simulink model "uav_simulation_tarot"  (R2020a)
settings: Solver=VariableStepAuto  StartTime=0.0  StopTime=sim_params.max_sim_time  FixedStep=uav.dynamics_srate  MaxStep=uav.dynamics_srate  MinStep=.01  RelTol=1e-3
undefined symbols (not defined in the file): deg, DiscIntNeverNeededParam, processes, rad, s, sim_params, trajectory, uav
libraries: aerolibconvert2 x2, shared6dof x1
(part 1 of 2)
settings Model: Creator=Researcher  LastModifiedBy=darrahts
settings DataIOCC: ReturnWorkspaceOutputs=off
settings DebuggingCC: ArithmeticOperatorsInVariantConditions=warning
settings SFSimCC: SimUseLocalCustomCode=off  CustomCodeUndefinedFunction=UseInterfaceOnly
settings RTWCC: RTWUseLocalCustomCode=off

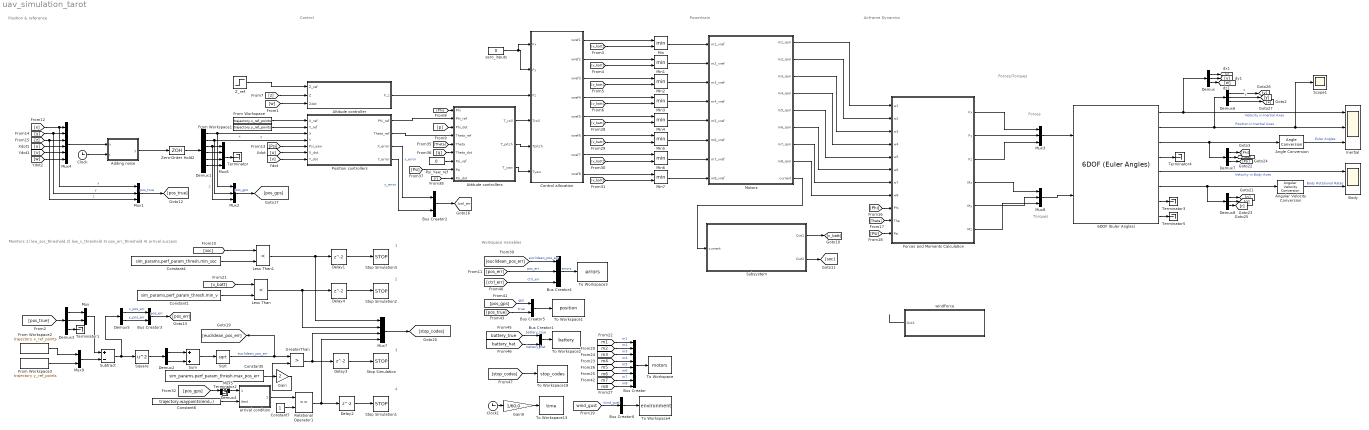
== system uav_simulation_tarot ==
  note: Airframe Dynamics
  note: 1
  note: Monitors
      | 	1) low_soc_threshold
      | 	2) low_v_threshold
      | 	3) pos_err_threshold
      | 	4) arrival success
  note: Powertrain
  note: Control
  note: 2
  note: 3
  note: 4
  note: Position & reference
  note: Workspace Variables
  note: Forces/Torques
  note: Torques
  note: Forces
  6DOF (Euler Angles) : shared6dof/6DOF (Euler Angles)  units=Metric (MKS)  mtype=Fixed  rep=Quaternion  xme_0=[sim_params.initial_conditions.X, sim_params.initial_conditions.Y, sim_params.initial_conditions.Z]  Vm_0=[0 0 0]  eul_0=[0 0 0]  pm_0=[0 0 0]  mass_0=uav.mass  mass_e=0.5  mass_f=2.0  inertia=uav.airframe.Jb  inertia_e=eye(3)  inertia_f=2*eye(3)  k_quat=1.0  vre_flag=on  abi_flag=off  aMode=0  xme_statename=''  Vm_statename=''  eul_statename=''  quat_statename=''  pm_statename=''  mass_statename=''
      settings: SourceProductBaseCode=AE,PW,MT,VE,VP
  Adding noise : MATLAB Function  TreatAsAtomicUnit=on  SystemSampleTime=uav.dynamics_srate
  Altitude controller : Subsystem
  Angle Conversion : aerolibconvert2/Angle Conversion  IU=rad  OU=deg
  Angular Velocity Conversion : aerolibconvert2/Angular Velocity Conversion  IU=rad/s  OU=deg/s
  Attitude controllers : Subsystem
  Body : Scope  NumInputPorts=2
  Bus Creator : BusCreator  Inputs=8
  Bus Creator{1..3,5} (4 alike) : BusCreator  Inputs=2
  Bus Creator4 : BusCreator  Inputs=3
  Bus Creator6 : BusCreator  Inputs=1
  Clock : Clock
  Clock1 : Clock
  Constant1 : Constant  Value=sim_params.perf_param_thresh.min_v
  Constant4 : Constant  Value=sim_params.perf_param_thresh.min_soc
  Constant5 : Constant  Value=sim_params.perf_param_thresh.max_pos_err
  Constant6 : Constant  Value=trajectory.waypoints(end,:)
  Constant7 : Constant
  Control allocation : MATLAB Function  TreatAsAtomicUnit=on
  Delay{1..4} (4 alike) : Delay
  Demux{,3..4,6..8} (6 alike) : Demux  Outputs=3
  Demux1 : Demux  Outputs=6
  Demux2 : Demux  Outputs=2
  Demux5 : Demux  Outputs=2
  Forces and Moments Calculation : MATLAB Function  TreatAsAtomicUnit=on
  From Workspace : FromWorkspace  VariableName=trajectory.x_ref_points  SampleTime=trajectory.sample_time
  From Workspace1 : FromWorkspace  VariableName=trajectory.y_ref_points  SampleTime=trajectory.sample_time
  From Workspace2 : FromWorkspace  VariableName=trajectory.x_ref_points  SampleTime=trajectory.sample_time
  From Workspace3 : FromWorkspace  VariableName=trajectory.y_ref_points  SampleTime=trajectory.sample_time
  Gain : Gain  Gain=2
  Gain9 : Gain  Gain=1/60.0
  GreaterThan : RelationalOperator  Operator=>  OutDataTypeStr=boolean  RndMeth=Simplest
  Inertial : Scope  NumInputPorts=3
  Less Than : RelationalOperator  Operator=<  OutDataTypeStr=boolean  RndMeth=Simplest
  Less Than1 : RelationalOperator  Operator=<  OutDataTypeStr=boolean  RndMeth=Simplest
  Min{,1..7} (8 alike) : MinMax  Inputs=2
  Motors : Subsystem
  Mux : Mux  Inputs=2
  Mux{1..3,8} (4 alike) : Mux  Inputs=3
  Mux4 : Mux  Inputs=6
  Mux5 : Mux  Inputs=2
  Mux6 : Mux
  Mux7 : Mux
  Mux9 : Mux  Inputs=2
  Position controllers : Subsystem
  Psi_Yaw_ref : Constant  Value=0
  Relational Operator1 : RelationalOperator  Operator===  OutDataTypeStr=boolean  RndMeth=Simplest
  Scope1 : Scope
  Sqrt : Sqrt  SaturateOnIntegerOverflow=on
  Square : Math  Operator=square  SaturateOnIntegerOverflow=on
  Stop Simulation{,1..3} (4 alike) : Stop
  Subsystem : Subsystem
  Subtract : Sum  Inputs=+-
  Sum : Sum
  Terminator{,1..5} (6 alike) : Terminator
  To Workspace : ToWorkspace  VariableName=motors  SaveFormat=Timeseries  SampleTime=-1
  To Workspace1 : ToWorkspace  VariableName=position  SaveFormat=Timeseries  SampleTime=-1
  To Workspace13 : ToWorkspace  VariableName=time  SaveFormat=Timeseries  SampleTime=-1
  To Workspace18 : ToWorkspace  VariableName=stop_codes  SaveFormat=Timeseries  SampleTime=-1
  To Workspace2 : ToWorkspace  VariableName=battery  SaveFormat=Timeseries  SampleTime=-1
  To Workspace3 : ToWorkspace  VariableName=errors  SaveFormat=Timeseries  SampleTime=-1
  To Workspace4 : ToWorkspace  VariableName=environment  SaveFormat=Timeseries  SampleTime=-1
  Z_ref : Step  Before=3  After=3  SampleTime=0
  Zero-Order Hold2 : ZeroOrderHold  SampleTime=uav.dynamics_srate
  arrival condition : MATLAB Function  TreatAsAtomicUnit=on
  windForce : Subsystem
  zero_inputs : Constant  Value=0
  wires:
  Clock/1 -> Adding noise/2(t)
  [y] -> Mux1/2, Mux4/2  "y"
  Zero-Order Hold2/1 -> Demux1/1
  [x] -> Mux1/1, Mux4/1  "x"
  [w] -> Mux4/6
  [z] -> Mux1/3, Mux4/3  "z"
  [v] -> Mux4/5
  [u] -> Mux4/4
  Mux4/1 -> Adding noise/1(u)
  Demux1/3 -> Mux2/3, Mux6/1  "z"
  Demux1/5 -> Mux6/3
  Demux1/4 -> Mux6/2
  Demux1/6 -> Mux6/4
  Demux1/2 -> Position controllers/4(Y), Mux2/2  "y"
  Demux1/1 -> Position controllers/3(X), Mux2/1  "x"
  Control allocation/6(wref6) -> Min5/1
  [v_batt] -> Min4/2
  Attitude controllers/1(T_roll) -> Control allocation/4(Troll)
  Min3/1 -> Motors/4(m4_vref)
  Position controllers/1(Phi_ref) -> Attitude controllers/2(Phi_ref)
  [r] -> Attitude controllers/9(Psi_dot)
  Z_ref/1 -> Altitude controller/1(Z_ref)
  [v_batt] -> Min3/2
  [v_batt] -> Min7/2
  Attitude controllers/3(T_yaw) -> Control allocation/6(Tyaw)
  Control allocation/8(wref8) -> Min7/1
  Bus Creator2/1 -> [ctrl_err]
  Min7/1 -> Motors/8(m8_vref)
  [Psi] -> Position controllers/5(Psi_yaw)
  [w] -> Altitude controller/3(Zdot)
  [u] -> Position controllers/6(X_dot)
  From Workspace/1 -> Position controllers/1(X_ref)
  Control allocation/7(wref7) -> Min6/1
  Position controllers/3(X_error) -> Bus Creator2/1  "x_error"
  Min2/1 -> Motors/3(m3_vref)
  Control allocation/3(wref3) -> Min2/1
  Min4/1 -> Motors/5(m5_vref)
  Attitude controllers/2(T_pitch) -> Control allocation/5(Tpitch)
  [Theta] -> Attitude controllers/5(Theta)
  Position controllers/2(Theta_ref) -> Attitude controllers/4(Theta_ref)
  Control allocation/1(wref1) -> Min/1
  Altitude controller/1(F_z) -> Control allocation/3(Fz)
  [Phi] -> Attitude controllers/1(Phi)
  [z] -> Altitude controller/2(Z)
  Position controllers/4(Y_error) -> Bus Creator2/2  "y_error"
  [v_batt] -> Min6/2
  Min5/1 -> Motors/6(m6_vref)
  Control allocation/4(wref4) -> Min3/1
  Min1/1 -> Motors/2(m2_vref)
  Control allocation/5(wref5) -> Min4/1
  Control allocation/2(wref2) -> Min1/1
  From Workspace1/1 -> Position controllers/2(Y_ref)
  [v] -> Position controllers/7(Y_dot)
  [Psi] -> Attitude controllers/8(Psi)
  Min6/1 -> Motors/7(m7_vref)
  zero_inputs/1 -> Control allocation/2(Fy), Control allocation/1(Fx)
  Min/1 -> Motors/1(m1_vref)
  [v_batt] -> Min/2
  [q] -> Attitude controllers/6(Theta_dot)
  Psi_Yaw_ref/1 -> Attitude controllers/7(Psi_ref)
  [p] -> Attitude controllers/3(Phi_dot)
  [v_batt] -> Min5/2
  [v_batt] -> Min1/2
  [v_batt] -> Min2/2
  Constant7/1 -> Relational Operator1/2
  Mux7/1 -> [stop_codes]
  Constant6/1 -> arrival condition/2(dest)
  Demux2/2 -> Sum/2
  Delay2/1 -> Stop Simulation1/1
  Constant5/1 -> Gain/1
  Gain9/1 -> To Workspace13/1
  arrival condition/1(arrived) -> Relational Operator1/1
  Demux2/1 -> Sum/1
  [pos_true] -> Demux3/1
  Mux9/1 -> Subtract/2
  Delay1/1 -> Stop Simulation3/1
  From Workspace3/1 -> Mux9/2
  Constant4/1 -> Less Than1/2
  Clock1/1 -> Gain9/1
  Sum/1 -> Sqrt/1
  [soc] -> Less Than1/1
  GreaterThan/1 -> Mux7/3, Delay3/1
  Sqrt/1 -> [euclidean_pos_err], GreaterThan/1  "euclidean_pos_err"
  Square/1 -> Demux2/1
  Subtract/1 -> Demux5/1, Square/1
  From Workspace2/1 -> Mux9/1
  [pos_gps] -> Demux4/1
  Relational Operator1/1 -> Mux7/4, Delay2/1
  Delay3/1 -> Stop Simulation/1
  Less Than1/1 -> Delay1/1, Mux7/1
  [stop_codes] -> To Workspace18/1
  [pos_gps] -> Bus Creator5/1  "gps"
  [battery_true] -> Bus Creator1/1  "battery_true"
  [battery_hat] -> Bus Creator1/2  "battery_hat"
  Motors/9(current) -> Subsystem/1(current)
  Subsystem/1(Out1) -> [v_batt]
  Subsystem/2(Out2) -> [soc]
  windForce/1(Out1) -> ?
  [m2] -> Bus Creator/2  "m2"
  Adding noise/1(y) -> Zero-Order Hold2/1
  Mux1/1 -> [pos_true]  "pos_true"
  Constant1/1 -> Less Than/2
  [v_batt] -> Less Than/1
  Delay4/1 -> Stop Simulation2/1
  Less Than/1 -> Mux7/2, Delay4/1
  [m1] -> Bus Creator/1  "m1"
  Bus Creator/1 -> To Workspace/1
  [m3] -> Bus Creator/3  "m3"
  [m4] -> Bus Creator/4  "m4"
  [m5] -> Bus Creator/5  "m5"
  [m6] -> Bus Creator/6  "m6"
  [m7] -> Bus Creator/7  "m7"
  [m8] -> Bus Creator/8  "m8"
  [pos_true] -> Bus Creator5/2  "true"
  Demux3/1 -> Mux/1
  Demux3/2 -> Mux/2
  Mux/1 -> Subtract/1
  Mux6/1 -> Terminator/1
  Mux2/1 -> [pos_gps]  "pos_gps"
  Demux3/3 -> Terminator1/1
  Demux4/1 -> Mux5/1
  Demux4/2 -> Mux5/2
  Mux5/1 -> arrival condition/1(currentpos)
  Demux4/3 -> Terminator2/1
  Bus Creator1/1 -> To Workspace2/1
  Demux5/1 -> Bus Creator3/1  "x_pos_err"
  Demux5/2 -> Bus Creator3/2  "y_pos_err"
  Bus Creator3/1 -> [pos_err]  "pos_err"
  [euclidean_pos_err] -> Bus Creator4/1  "euclidean_pos_err"
  [ctrl_err] -> Bus Creator4/3  "ctrl_err"
  [pos_err] -> Bus Creator4/2  "pos_err"
  Bus Creator4/1 -> To Workspace3/1  "errors"
  Bus Creator5/1 -> To Workspace1/1
  [wind_gust] -> Bus Creator6/1  "wind_gust"
  Bus Creator6/1 -> To Workspace4/1
  Gain/1 -> GreaterThan/2
  Forces and Moments Calculation/3(Fz) -> Mux3/3
  Forces and Moments Calculation/6(Mz) -> Mux8/3
  Angle Conversion/1 -> Inertial/3  "Euler Angles"
  Mux3/1 -> 6DOF (Euler Angles)/1
  Forces and Moments Calculation/5(My) -> Mux8/2
  Angular Velocity Conversion/1 -> Body/2  "Body Rotational Rates"
  Forces and Moments Calculation/2(Fy) -> Mux3/2
  Demux6/2 -> [y]  "y"
  Mux8/1 -> 6DOF (Euler Angles)/2
  6DOF (Euler Angles)/2 -> Demux6/1, Scope1/1, Inertial/2  "Position in Inertial Axes"
  Demux8/1 -> [p]
  Demux/3 -> [w]
  6DOF (Euler Angles)/8 -> Terminator5/1
  Demux6/1 -> [x]  "x"
  Demux7/2 -> [Theta]
  Forces and Moments Calculation/4(Mx) -> Mux8/1
  6DOF (Euler Angles)/7 -> Terminator3/1
  6DOF (Euler Angles)/6 -> Demux8/1, Angular Velocity Conversion/1
  Demux8/3 -> [r]
  Demux7/1 -> [Phi]
  Demux8/2 -> [q]
  6DOF (Euler Angles)/3 -> Demux7/1, Angle Conversion/1
  6DOF (Euler Angles)/4 -> Terminator4/1
  6DOF (Euler Angles)/1 -> Demux/1, Inertial/1  "Velocity in Inertial Axes"
  Demux6/3 -> [z]
  Forces and Moments Calculation/1(Fx) -> Mux3/1
  6DOF (Euler Angles)/5 -> Body/1  "Velocity in Body Axes"
  Demux7/3 -> [Psi]
  Demux/2 -> [v]
  Demux/1 -> [u]
  Motors/1(m1_rpm) -> Forces and Moments Calculation/1(w1)
  Motors/2(m2_rpm) -> Forces and Moments Calculation/2(w2)
  Motors/3(m3_rpm) -> Forces and Moments Calculation/3(w3)
  Motors/4(m4_rpm) -> Forces and Moments Calculation/4(w4)
  Motors/5(m5_rpm) -> Forces and Moments Calculation/5(w5)
  Motors/6(m6_rpm) -> Forces and Moments Calculation/6(w6)
  Motors/7(m7_rpm) -> Forces and Moments Calculation/7(w7)
  Motors/8(m8_rpm) -> Forces and Moments Calculation/8(w8)
  [Psi] -> Forces and Moments Calculation/11(Psi)
  [Theta] -> Forces and Moments Calculation/10(The)
  [Phi] -> Forces and Moments Calculation/9(Phi)

== system uav_simulation_tarot/Altitude controller ==
  Z_ref : Inport
  Z : Inport  Port=2
  Zdot : Inport  Port=3
  Add : Sum  Inputs=+++
  Add2 : Sum  Inputs=+-
  Constant2 : Constant  Value=9.8*uav.mass
  Kdz : Gain  Gain=-1
  Kpz : Gain  Gain=-0.5
  mass : Gain  Gain=uav.mass
  mass1 : Gain  Gain=uav.mass
  F_z : Outport  VectorParamsAs1DForOutWhenUnconnected=off
  wires:
  Add2/1 -> Kpz/1
  Constant2/1 -> Add/1
  Z/1 -> Add2/1
  Add/1 -> F_z/1
  Z_ref/1 -> Add2/2
  Zdot/1 -> Kdz/1
  Kpz/1 -> mass/1
  Kdz/1 -> mass1/1
  mass1/1 -> Add/3
  mass/1 -> Add/2

== system uav_simulation_tarot/Attitude controllers ==
  Phi : Inport
  Phi_ref : Inport  Port=2
  Phi_dot : Inport  Port=3
  Theta_ref : Inport  Port=4
  Theta : Inport  Port=5
  Theta_dot : Inport  Port=6
  Psi_ref : Inport  Port=7
  Psi : Inport  Port=8
  Psi_dot : Inport  Port=9
  PD_pitch : Subsystem
  PD_roll : Subsystem
  PD_yaw : Subsystem
  T_roll : Outport  VectorParamsAs1DForOutWhenUnconnected=off
  T_pitch : Outport  Port=2  VectorParamsAs1DForOutWhenUnconnected=off
  T_yaw : Outport  Port=3  VectorParamsAs1DForOutWhenUnconnected=off
  wires:
  PD_yaw/1(Tyaw) -> T_yaw/1
  PD_roll/1(Troll) -> T_roll/1
  Theta_ref/1 -> PD_pitch/1(Theta_ref)
  Theta_dot/1 -> PD_pitch/3(Theta_dot)
  PD_pitch/1(Tpitch) -> T_pitch/1
  Phi/1 -> PD_roll/2(Phi)
  Psi_dot/1 -> PD_yaw/3(Psi_dot)
  Psi_ref/1 -> PD_yaw/1(Psi_ref)
  Theta/1 -> PD_pitch/2(Theta)
  Phi_dot/1 -> PD_roll/3(Phi_dot)
  Psi/1 -> PD_yaw/2(Psi)
  Phi_ref/1 -> PD_roll/1(Phi_ref)

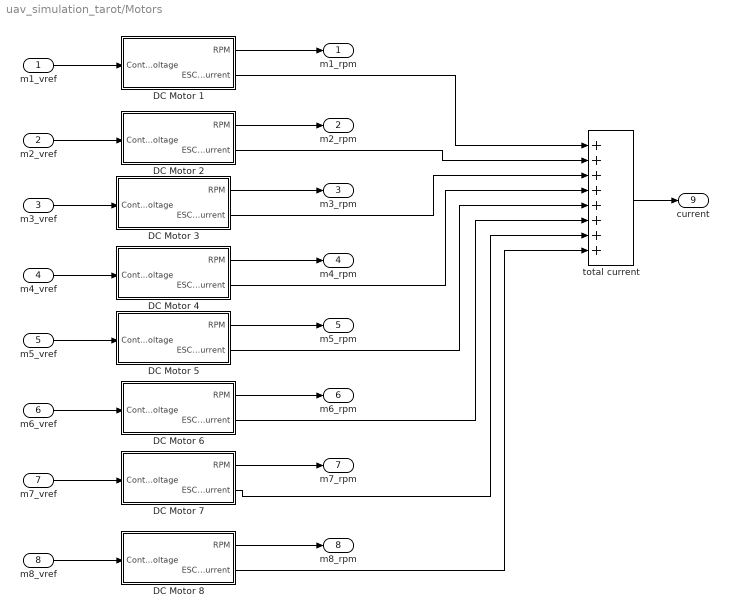
== system uav_simulation_tarot/Motors ==
  m1_vref : Inport
  m2_vref : Inport  Port=2
  m3_vref : Inport  Port=3
  m4_vref : Inport  Port=4
  m5_vref : Inport  Port=5
  m6_vref : Inport  Port=6
  m7_vref : Inport  Port=7
  m8_vref : Inport  Port=8
  DC Motor 1 : Subsystem
  DC Motor 2 : Subsystem
  DC Motor 3 : Subsystem
  DC Motor 4 : Subsystem
  DC Motor 5 : Subsystem
  DC Motor 6 : Subsystem
  DC Motor 7 : Subsystem
  DC Motor 8 : Subsystem
  total current : Sum  Inputs=++++++++
  m1_rpm : Outport  VectorParamsAs1DForOutWhenUnconnected=off
  m2_rpm : Outport  Port=2  VectorParamsAs1DForOutWhenUnconnected=off
  m3_rpm : Outport  Port=3  VectorParamsAs1DForOutWhenUnconnected=off
  m4_rpm : Outport  Port=4  VectorParamsAs1DForOutWhenUnconnected=off
  m5_rpm : Outport  Port=5  VectorParamsAs1DForOutWhenUnconnected=off
  m6_rpm : Outport  Port=6  VectorParamsAs1DForOutWhenUnconnected=off
  m7_rpm : Outport  Port=7  VectorParamsAs1DForOutWhenUnconnected=off
  m8_rpm : Outport  Port=8  VectorParamsAs1DForOutWhenUnconnected=off
  current : Outport  Port=9  VectorParamsAs1DForOutWhenUnconnected=off
  wires:
  DC Motor 6/2(ESC Current) -> total current/6
  DC Motor 7/2(ESC Current) -> total current/7
  DC Motor 5/2(ESC Current) -> total current/5
  DC Motor 8/2(ESC Current) -> total current/8
  DC Motor 1/2(ESC Current) -> total current/1
  DC Motor 2/2(ESC Current) -> total current/2
  DC Motor 4/2(ESC Current) -> total current/4
  DC Motor 3/2(ESC Current) -> total current/3
  DC Motor 5/1(RPM) -> m5_rpm/1
  DC Motor 7/1(RPM) -> m7_rpm/1
  DC Motor 2/1(RPM) -> m2_rpm/1
  DC Motor 3/1(RPM) -> m3_rpm/1
  DC Motor 4/1(RPM) -> m4_rpm/1
  DC Motor 6/1(RPM) -> m6_rpm/1
  DC Motor 8/1(RPM) -> m8_rpm/1
  DC Motor 1/1(RPM) -> m1_rpm/1
  m1_vref/1 -> DC Motor 1/1(Control  Voltage)
  m7_vref/1 -> DC Motor 7/1(Control  Voltage)
  m8_vref/1 -> DC Motor 8/1(Control  Voltage)
  m6_vref/1 -> DC Motor 6/1(Control  Voltage)
  m5_vref/1 -> DC Motor 5/1(Control  Voltage)
  m4_vref/1 -> DC Motor 4/1(Control  Voltage)
  m3_vref/1 -> DC Motor 3/1(Control  Voltage)
  m2_vref/1 -> DC Motor 2/1(Control  Voltage)
  total current/1 -> current/1

== system uav_simulation_tarot/Position controllers ==
  X_ref : Inport
  Y_ref : Inport  Port=2
  X : Inport  Port=3
  Y : Inport  Port=4
  Psi_yaw : Inport  Port=5
  X_dot : Inport  Port=6
  Y_dot : Inport  Port=7
  Error Rotations : Subsystem
  PD_Phi_des : Subsystem
  PD_Theta_des : Subsystem
  Phi_ref : Outport  VectorParamsAs1DForOutWhenUnconnected=off
  Theta_ref : Outport  Port=2  VectorParamsAs1DForOutWhenUnconnected=off
  X_error : Outport  Port=3  VectorParamsAs1DForOutWhenUnconnected=off
  Y_error : Outport  Port=4  VectorParamsAs1DForOutWhenUnconnected=off
  wires:
  Y/1 -> Error Rotations/4(Y)
  Y_ref/1 -> Error Rotations/2(Y_cmd)
  Error Rotations/4("Y error ") -> Y_error/1
  Error Rotations/3(X error) -> X_error/1
  Error Rotations/1(X Error in body Frame) -> PD_Theta_des/1(Xdot_ref)
  X/1 -> Error Rotations/3(X)
  Y_dot/1 -> PD_Phi_des/2(Ydot)
  PD_Phi_des/1(Phi_des) -> Phi_ref/1
  Error Rotations/2(Y Error in Body Frame) -> PD_Phi_des/1(Ydot_ref)
  Psi_yaw/1 -> Error Rotations/5(Psi)
  PD_Theta_des/1(Theta_des) -> Theta_ref/1
  X_dot/1 -> PD_Theta_des/2(Xdot)
  X_ref/1 -> Error Rotations/1(X_cmd)

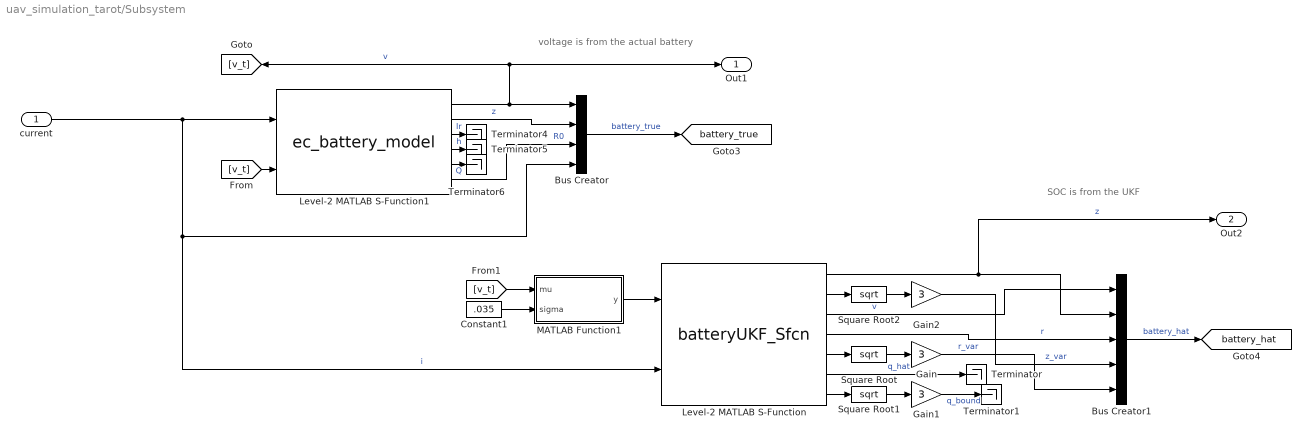
== system uav_simulation_tarot/Subsystem ==
  note: SOC is from the UKF
  note: voltage is from the actual battery
  current : Inport
  Bus Creator : BusCreator  Inputs=4
  Bus Creator1 : BusCreator  Inputs=5
  Constant1 : Constant  Value=.035
  Gain : Gain  Gain=3
  Gain1 : Gain  Gain=3
  Gain2 : Gain  Gain=3
  Level-2 MATLAB S-Function : M-S-Function  FunctionName=batteryUKF_Sfcn  Parameters=uav.battery, uav.battery.dt, sim_params.battery_estimator
      mask Display:
      | port_label('input', 1, 'voltage');
      | port_label('input', 2, 'current');
      | port_label('output', 1, 'soc_hat');
      | port_label('output', 2, 'soc_bound');
      | port_label('output', 3, 'voltage_hat');
      | port_label('output', 4, 'r0_hat');
      | port_label('output', 5, 'r0_bound');
      | port_label('output', 6, 'q_hat');
      | port_label('output', 7, 'q_bound');
      | 
      | disp("UKF");
  Level-2 MATLAB S-Function1 : M-S-Function  FunctionName=ec_battery_model  Parameters=uav.battery
      mask Display:
      | port_label('output', 1, 'v');
      | port_label('output', 2, 'z');
      | port_label('output', 3, 'Ir');
      | port_label('output', 4, 'h');
      | port_label('output', 5, 'Q');
      | port_label('output', 6, 'R0');
      | 
      | port_label('input', 1, 'u');
      | port_label('input', 2, 'v_(t-1)');
  MATLAB Function1 : MATLAB Function  TreatAsAtomicUnit=on
  Square Root : Sqrt  SaturateOnIntegerOverflow=on
  Square Root1 : Sqrt  SaturateOnIntegerOverflow=on
  Square Root2 : Sqrt  SaturateOnIntegerOverflow=on
  Terminator{,1,4..6} (5 alike) : Terminator
  Out1 : Outport
  Out2 : Outport  Port=2
  tag scope: battery_hat=global, battery_true=global
  wires:
  MATLAB Function1/1(y) -> Level-2 MATLAB S-Function/1
  Constant1/1 -> MATLAB Function1/2(sigma)
  Level-2 MATLAB S-Function/5 -> Square Root/1
  Square Root/1 -> Gain/1
  Bus Creator/1 -> [battery_true]  "battery_true"
  Square Root1/1 -> Gain1/1
  Square Root2/1 -> Gain2/1
  Level-2 MATLAB S-Function/2 -> Square Root2/1
  Level-2 MATLAB S-Function/7 -> Square Root1/1
  Level-2 MATLAB S-Function/3 -> Bus Creator1/1  "v"
  Level-2 MATLAB S-Function/1 -> Bus Creator1/2, Out2/1  "z"
  Gain2/1 -> Bus Creator1/4  "z_var"
  Level-2 MATLAB S-Function/4 -> Bus Creator1/3  "r"
  Gain/1 -> Bus Creator1/5  "r_var"
  Gain1/1 -> Terminator1/1  "q_bound"
  Bus Creator1/1 -> [battery_hat]  "battery_hat"
  current/1 -> Level-2 MATLAB S-Function/2, Bus Creator/4, Level-2 MATLAB S-Function1/1  "i"
  Level-2 MATLAB S-Function/6 -> Terminator/1  "q_hat"
  Level-2 MATLAB S-Function1/3 -> Terminator4/1  "Ir"
  Level-2 MATLAB S-Function1/4 -> Terminator5/1  "h"
  Level-2 MATLAB S-Function1/5 -> Terminator6/1  "Q"
  [v_t] -> Level-2 MATLAB S-Function1/2
  Level-2 MATLAB S-Function1/1 -> Out1/1, [v_t], Bus Creator/1  "v"
  Level-2 MATLAB S-Function1/2 -> Bus Creator/2  "z"
  Level-2 MATLAB S-Function1/6 -> Bus Creator/3  "R0"
  [v_t] -> MATLAB Function1/1(mu)

== system uav_simulation_tarot/windForce ==
  Constant10 : Constant  Value=[0;0;0]
  Gain : Gain  Gain=2
  Manual Switch1 : ManualSwitch  CurrentSetting=0
  Mux9 : Mux  Inputs=3
  Random Number : RandomNumber  Mean=processes.environment.wind.gust(1)  Variance=processes.environment.wind.gust(2)  Seed=37  SampleTime=uav.dynamics_srate
  Random Number1 : RandomNumber  Mean=processes.environment.wind.gust(1)  Variance=processes.environment.wind.gust(2)  Seed=41  SampleTime=uav.dynamics_srate
  Random Number2 : RandomNumber  Mean=processes.environment.wind.gust(1)  Variance=processes.environment.wind.gust(2)  SampleTime=uav.dynamics_srate
  Out1 : Outport
  tag scope: wind_gust=global
  wires:
  Random Number1/1 -> Mux9/2
  Mux9/1 -> Gain/1
  Manual Switch1/1 -> [wind_gust], Out1/1
  Random Number2/1 -> Mux9/3
  Random Number/1 -> Mux9/1
  Constant10/1 -> Manual Switch1/1
  Gain/1 -> Manual Switch1/2

== system uav_simulation_tarot/Attitude controllers/PD_pitch ==
  Theta_ref : Inport
  Theta : Inport  Port=2
  Theta_dot : Inport  Port=3
  Add : Sum  Inputs=-+
  Gain : Gain  Gain=3
  Gain1 : Gain
  Gain2 : Gain  Gain=-1
  Sum : Sum  Inputs=|++
  Tpitch : Outport  VectorParamsAs1DForOutWhenUnconnected=off
  wires:
  Gain2/1 -> Tpitch/1
  Gain/1 -> Sum/1
  Theta/1 -> Add/2
  Add/1 -> Gain/1
  Gain1/1 -> Sum/2
  Sum/1 -> Gain2/1
  Theta_dot/1 -> Gain1/1
  Theta_ref/1 -> Add/1

== system uav_simulation_tarot/Attitude controllers/PD_roll ==
  Phi_ref : Inport
  Phi : Inport  Port=2
  Phi_dot : Inport  Port=3
  Add : Sum  Inputs=-+
  Gain : Gain  Gain=3
  Gain1 : Gain
  Gain2 : Gain  Gain=-1
  Sum : Sum  Inputs=|++
  Troll : Outport  VectorParamsAs1DForOutWhenUnconnected=off
  wires:
  Phi_ref/1 -> Add/1
  Phi_dot/1 -> Gain1/1
  Sum/1 -> Gain2/1
  Gain1/1 -> Sum/2
  Add/1 -> Gain/1
  Phi/1 -> Add/2
  Gain/1 -> Sum/1
  Gain2/1 -> Troll/1

== system uav_simulation_tarot/Attitude controllers/PD_yaw ==
  Psi_ref : Inport
  Psi : Inport  Port=2
  Psi_dot : Inport  Port=3
  Add : Sum  Inputs=-+
  Gain : Gain  Gain=3
  Gain1 : Gain
  Gain2 : Gain  Gain=-1
  Sum : Sum  Inputs=|++
  Tyaw : Outport  VectorParamsAs1DForOutWhenUnconnected=off
  wires:
  Psi_ref/1 -> Add/1
  Psi_dot/1 -> Gain1/1
  Sum/1 -> Gain2/1
  Gain1/1 -> Sum/2
  Add/1 -> Gain/1
  Psi/1 -> Add/2
  Gain/1 -> Sum/1
  Gain2/1 -> Tyaw/1

== system uav_simulation_tarot/Motors/DC Motor 1 ==
  Control  Voltage : Inport
  Bus Creator : BusCreator  Inputs=3
  Electrical part : Subsystem
  Mechanical part : Subsystem
  Scope : Scope
  StaticTfric : Constant  Value=0
  RPM : Outport  VectorParamsAs1DForOutWhenUnconnected=off
  ESC Current : Outport  Port=2  VectorParamsAs1DForOutWhenUnconnected=off
  tag scope: m1=global
  wires:
  StaticTfric/1 -> Mechanical part/2(Static Friction Torque)
  Control  Voltage/1 -> Electrical part/1(ESC voltage)
  Bus Creator/1 -> [m1]  "m1"
  Mechanical part/1(rpm) -> RPM/1, Bus Creator/1  "rpm"
  Electrical part/1(Electrical Torque) -> Mechanical part/1(Electrical Torque)  "torque"
  Electrical part/2(current) -> ESC Current/1, Bus Creator/3  "current"
  Mechanical part/2(torque) -> Scope/1, Bus Creator/2  "torque"
  Mechanical part/3(angular_speed) -> Electrical part/2(w angular speed)

== system uav_simulation_tarot/Motors/DC Motor 2 ==
  Control  Voltage : Inport
  Bus Creator : BusCreator  Inputs=3
  Electrical part : Subsystem
  Mechanical part : Subsystem
  StaticTfric : Constant  Value=0
  RPM : Outport  VectorParamsAs1DForOutWhenUnconnected=off
  ESC Current : Outport  Port=2  VectorParamsAs1DForOutWhenUnconnected=off
  tag scope: m2=global
  wires:
  StaticTfric/1 -> Mechanical part/2(Static Friction Torque)
  Control  Voltage/1 -> Electrical part/1(ESC voltage)
  Bus Creator/1 -> [m2]  "m2"
  Mechanical part/1(rpm) -> RPM/1, Bus Creator/1  "rpm"
  Electrical part/1(Electrical Torque) -> Mechanical part/1(Electrical Torque)  "torque"
  Electrical part/2(current) -> ESC Current/1, Bus Creator/3  "current"
  Mechanical part/2(torque) -> Bus Creator/2  "torque"
  Mechanical part/3(angular_velocity) -> Electrical part/2(w angular speed)

== system uav_simulation_tarot/Motors/DC Motor 3 ==
  Control  Voltage : Inport
  Bus Creator : BusCreator  Inputs=3
  Electrical part : Subsystem
  Mechanical part : Subsystem
  StaticTfric : Constant  Value=0
  RPM : Outport  VectorParamsAs1DForOutWhenUnconnected=off
  ESC Current : Outport  Port=2  VectorParamsAs1DForOutWhenUnconnected=off
  tag scope: m3=global
  wires:
  StaticTfric/1 -> Mechanical part/2(Static Friction Torque)
  Control  Voltage/1 -> Electrical part/1(ESC voltage)
  Bus Creator/1 -> [m3]  "m3"
  Mechanical part/1(rpm) -> RPM/1, Bus Creator/1  "rpm"
  Electrical part/1(Electrical Torque) -> Mechanical part/1(Electrical Torque)  "torque"
  Electrical part/2(current) -> ESC Current/1, Bus Creator/3  "current"
  Mechanical part/2(torque) -> Bus Creator/2  "torque"
  Mechanical part/3(angular_velocity) -> Electrical part/2(w angular speed)

== system uav_simulation_tarot/Motors/DC Motor 4 ==
  Control  Voltage : Inport
  Bus Creator : BusCreator  Inputs=3
  Electrical part : Subsystem
  Mechanical part : Subsystem
  StaticTfric : Constant  Value=0
  RPM : Outport  VectorParamsAs1DForOutWhenUnconnected=off
  ESC Current : Outport  Port=2  VectorParamsAs1DForOutWhenUnconnected=off
  tag scope: m4=global
  wires:
  StaticTfric/1 -> Mechanical part/2(Static Friction Torque)
  Control  Voltage/1 -> Electrical part/1(ESC voltage)
  Bus Creator/1 -> [m4]  "m4"
  Mechanical part/1(rpm) -> RPM/1, Bus Creator/1  "rpm"
  Electrical part/1(Electrical Torque) -> Mechanical part/1(Electrical Torque)  "torque"
  Electrical part/2(current) -> ESC Current/1, Bus Creator/3  "current"
  Mechanical part/2(torque) -> Bus Creator/2  "torque"
  Mechanical part/3(angular_velocity) -> Electrical part/2(w angular speed)

== system uav_simulation_tarot/Motors/DC Motor 5 ==
  Control  Voltage : Inport
  Bus Creator : BusCreator  Inputs=3
  Electrical part : Subsystem
  Mechanical part : Subsystem
  StaticTfric : Constant  Value=0
  RPM : Outport  VectorParamsAs1DForOutWhenUnconnected=off
  ESC Current : Outport  Port=2  VectorParamsAs1DForOutWhenUnconnected=off
  tag scope: m5=global
  wires:
  StaticTfric/1 -> Mechanical part/2(Static Friction Torque)
  Control  Voltage/1 -> Electrical part/1(ESC voltage)
  Bus Creator/1 -> [m5]  "m5"
  Mechanical part/1(rpm) -> RPM/1, Bus Creator/1  "rpm"
  Electrical part/1(Electrical Torque) -> Mechanical part/1(Electrical Torque)  "torque"
  Electrical part/2(current) -> ESC Current/1, Bus Creator/3  "current"
  Mechanical part/2(torque) -> Bus Creator/2  "torque"
  Mechanical part/3(angular_velocity) -> Electrical part/2(w angular speed)

== system uav_simulation_tarot/Motors/DC Motor 6 ==
  Control  Voltage : Inport
  Bus Creator : BusCreator  Inputs=3
  Electrical part : Subsystem
  Mechanical part : Subsystem
  StaticTfric : Constant  Value=0
  RPM : Outport  VectorParamsAs1DForOutWhenUnconnected=off
  ESC Current : Outport  Port=2  VectorParamsAs1DForOutWhenUnconnected=off
  tag scope: m6=global
  wires:
  StaticTfric/1 -> Mechanical part/2(Static Friction Torque)
  Control  Voltage/1 -> Electrical part/1(ESC voltage)
  Bus Creator/1 -> [m6]  "m6"
  Mechanical part/1(rpm) -> RPM/1, Bus Creator/1  "rpm"
  Electrical part/1(Electrical Torque) -> Mechanical part/1(Electrical Torque)  "torque"
  Electrical part/2(current) -> ESC Current/1, Bus Creator/3  "current"
  Mechanical part/2(torque) -> Bus Creator/2  "torque"
  Mechanical part/3(angular_velocity) -> Electrical part/2(w angular speed)

== system uav_simulation_tarot/Motors/DC Motor 7 ==
  Control  Voltage : Inport
  Bus Creator : BusCreator  Inputs=3
  Electrical part : Subsystem
  Mechanical part : Subsystem
  StaticTfric : Constant  Value=0
  RPM : Outport  VectorParamsAs1DForOutWhenUnconnected=off
  ESC Current : Outport  Port=2  VectorParamsAs1DForOutWhenUnconnected=off
  tag scope: m7=global
  wires:
  StaticTfric/1 -> Mechanical part/2(Static Friction Torque)
  Control  Voltage/1 -> Electrical part/1(ESC voltage)
  Bus Creator/1 -> [m7]  "m7"
  Mechanical part/1(rpm) -> RPM/1, Bus Creator/1  "rpm"
  Electrical part/1(Electrical Torque) -> Mechanical part/1(Electrical Torque)  "torque"
  Electrical part/2(current) -> ESC Current/1, Bus Creator/3  "current"
  Mechanical part/2(torque) -> Bus Creator/2  "torque"
  Mechanical part/3(angular_velocity) -> Electrical part/2(w angular speed)

== system uav_simulation_tarot/Motors/DC Motor 8 ==
  Control  Voltage : Inport
  Bus Creator : BusCreator  Inputs=3
  Electrical part : Subsystem
  Mechanical part : Subsystem
  StaticTfric : Constant  Value=0
  RPM : Outport  VectorParamsAs1DForOutWhenUnconnected=off
  ESC Current : Outport  Port=2  VectorParamsAs1DForOutWhenUnconnected=off
  tag scope: m8=global
  wires:
  StaticTfric/1 -> Mechanical part/2(Static Friction Torque)
  Control  Voltage/1 -> Electrical part/1(ESC voltage)
  Bus Creator/1 -> [m8]  "m8"
  Mechanical part/1(rpm) -> RPM/1, Bus Creator/1  "rpm"
  Electrical part/1(Electrical Torque) -> Mechanical part/1(Electrical Torque)  "torque"
  Electrical part/2(current) -> ESC Current/1, Bus Creator/3  "current"
  Mechanical part/2(torque) -> Bus Creator/2  "torque"
  Mechanical part/3(angular_velocity) -> Electrical part/2(w angular speed)

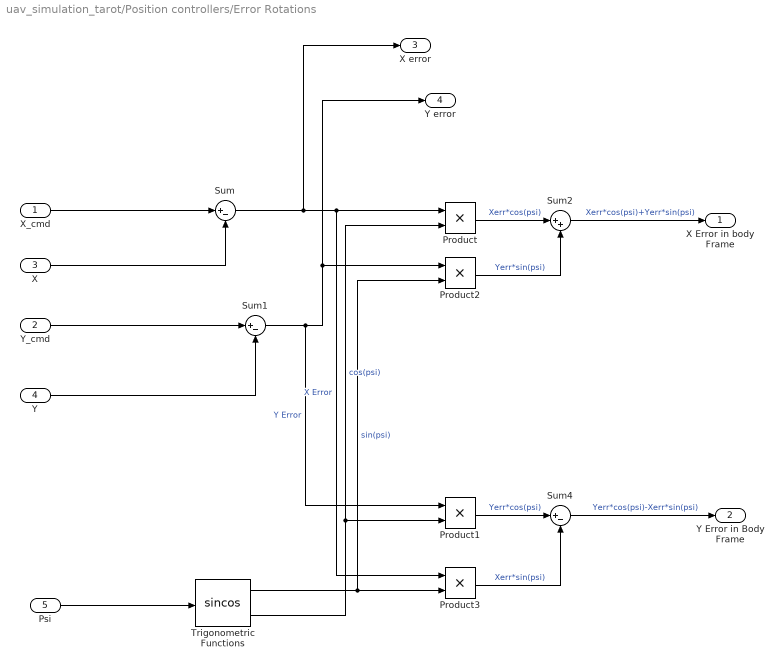
== system uav_simulation_tarot/Position controllers/Error Rotations ==
  X_cmd : Inport
  Y_cmd : Inport  Port=2
  X : Inport  Port=3
  Y : Inport  Port=4
  Psi : Inport  Port=5
  Product{,1..3} (4 alike) : Product
  Sum : Sum  Inputs=|+-
  Sum1 : Sum  Inputs=|+-
  Sum2 : Sum  Inputs=|++
  Sum4 : Sum  Inputs=|+-
  Trigonometric Functions : Trigonometry  Operator=sincos
  X Error in body Frame : Outport  VectorParamsAs1DForOutWhenUnconnected=off
  Y Error in Body Frame : Outport  Port=2  VectorParamsAs1DForOutWhenUnconnected=off
  X error : Outport  Port=3  VectorParamsAs1DForOutWhenUnconnected=off
  "Y error " : Outport  Port=4  VectorParamsAs1DForOutWhenUnconnected=off
  wires:
  Sum4/1 -> Y Error in Body Frame/1  "Yerr*cos(psi)-Xerr*sin(psi)"
  Product3/1 -> Sum4/2  "Xerr*sin(psi)"
  Sum1/1 -> "Y error "/1, Product2/1, Product1/1  "Y Error"
  Trigonometric Functions/1 -> Product2/2, Product3/2  "sin(psi)"
  Sum2/1 -> X Error in body Frame/1  "Xerr*cos(psi)+Yerr*sin(psi)"
  Y_cmd/1 -> Sum1/1
  X_cmd/1 -> Sum/1
  X/1 -> Sum/2
  Y/1 -> Sum1/2
  Sum/1 -> X error/1, Product3/1, Product/1  "X Error"
  Trigonometric Functions/2 -> Product/2, Product1/2  "cos(psi)"
  Product/1 -> Sum2/1  "Xerr*cos(psi)"
  Product2/1 -> Sum2/2  "Yerr*sin(psi)"
  Product1/1 -> Sum4/1  "Yerr*cos(psi)"
  Psi/1 -> Trigonometric Functions/1

== system uav_simulation_tarot/Position controllers/PD_Phi_des ==
  Ydot_ref : Inport
  Ydot : Inport  Port=2
  Add : Sum  Inputs=+-
  Gain : Gain  Gain=0.1
  Gain1 : Gain  Gain=0
  Gain2 : Gain  Gain=-1
  Saturation in radians : Saturate  UpperLimit=12*pi/180  LowerLimit=-12*pi/180
  Sum : Sum  Inputs=|+-
  Phi_des : Outport  VectorParamsAs1DForOutWhenUnconnected=off
  wires:
  Saturation in radians/1 -> Phi_des/1
  Ydot_ref/1 -> Add/1
  Ydot/1 -> Add/2, Gain1/1
  Gain1/1 -> Sum/2
  Add/1 -> Gain/1
  Gain/1 -> Sum/1
  Sum/1 -> Gain2/1
  Gain2/1 -> Saturation in radians/1

== system uav_simulation_tarot/Position controllers/PD_Theta_des ==
  Xdot_ref : Inport
  Xdot : Inport  Port=2
  Add : Sum  Inputs=+-
  Gain : Gain  Gain=0.1
  Gain1 : Gain  Gain=0
  Saturation in radians : Saturate  UpperLimit=12*pi/180  LowerLimit=-12*pi/180
  Sum : Sum  Inputs=|+-
  Theta_des : Outport  VectorParamsAs1DForOutWhenUnconnected=off
  wires:
  Sum/1 -> Saturation in radians/1
  Gain/1 -> Sum/1
  Add/1 -> Gain/1
  Gain1/1 -> Sum/2
  Xdot/1 -> Gain1/1, Add/2
  Xdot_ref/1 -> Add/1
  Saturation in radians/1 -> Theta_des/1

== system uav_simulation_tarot/Motors/DC Motor 1/Electrical part ==
  ESC voltage : Inport
  w angular speed : Inport  Port=2
  1/R : Gain  Gain=1/uav.motors(1).Req
  Ke (Torque constant)1 : Gain  Gain=uav.motors(1).Ke_eq
  Kt (Torque constant) Kt=Ke for an ideal square wave motor : Gain  Gain=uav.motors(1).Ke_eq
  Saturation : Saturate  UpperLimit=uav.motors(1).current_limit  LowerLimit=0
  Sum : Sum  Inputs=|+-
  Electrical Torque : Outport  VectorParamsAs1DForOutWhenUnconnected=off
  current : Outport  Port=2  VectorParamsAs1DForOutWhenUnconnected=off
  wires:
  1/R/1 -> Saturation/1  "current i"
  Sum/1 -> 1/R/1
  Kt (Torque constant) Kt=Ke for an ideal square wave motor/1 -> Electrical Torque/1
  Ke (Torque constant)1/1 -> Sum/2
  ESC voltage/1 -> Sum/1
  w angular speed/1 -> Ke (Torque constant)1/1
  Saturation/1 -> Kt (Torque constant) Kt=Ke for an ideal square wave motor/1, current/1

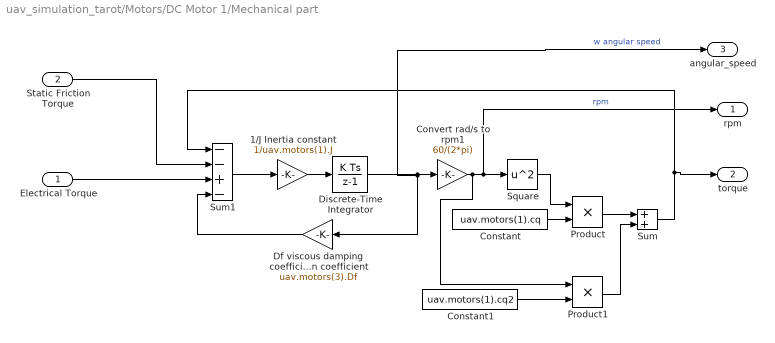
== system uav_simulation_tarot/Motors/DC Motor 1/Mechanical part ==
  Electrical Torque : Inport
  Static Friction Torque : Inport  Port=2
  1/J Inertia constant : Gain  Gain=1/uav.motors(1).J
  Constant : Constant  Value=uav.motors(1).cq
  Constant1 : Constant  Value=uav.motors(1).cq2
  Convert rad/s to rpm1 : Gain  Gain=60/(2*pi)
  "Df viscous damping coefficient Dynamic Friction coefficient " : Gain  Gain=uav.motors(3).Df
  Discrete-Time Integrator : DiscreteIntegrator  gainval=1  InitialCondition=sim_params.initial_conditions.w1  SampleTime=uav.dynamics_srate  ICPrevOutput=DiscIntNeverNeededParam  ICPrevScaledInput=DiscIntNeverNeededParam
  Product : Product
  Product1 : Product
  Square : Math  Operator=square  SaturateOnIntegerOverflow=on
  Sum : Sum
  Sum1 : Sum  Inputs=--+-
  rpm : Outport  VectorParamsAs1DForOutWhenUnconnected=off
  torque : Outport  Port=2
  angular_speed : Outport  Port=3
  wires:
  1/J Inertia constant/1 -> Discrete-Time Integrator/1
  Static Friction Torque/1 -> Sum1/2
  "Df viscous damping coefficient Dynamic Friction coefficient "/1 -> Sum1/4
  Discrete-Time Integrator/1 -> angular_speed/1, "Df viscous damping coefficient Dynamic Friction coefficient "/1, Convert rad/s to rpm1/1  "w angular speed"
  Sum1/1 -> 1/J Inertia constant/1
  Electrical Torque/1 -> Sum1/3
  Sum/1 -> torque/1, Sum1/1
  Square/1 -> Product/1
  Constant/1 -> Product/2
  Product/1 -> Sum/1
  Constant1/1 -> Product1/2
  Convert rad/s to rpm1/1 -> rpm/1, Square/1, Product1/1  "rpm"
  Product1/1 -> Sum/2

== system uav_simulation_tarot/Motors/DC Motor 2/Electrical part ==
  ESC voltage : Inport
  w angular speed : Inport  Port=2
  1/R : Gain  Gain=1/uav.motors(2).Req
  Ke (Torque constant)1 : Gain  Gain=uav.motors(2).Ke_eq
  Kt (Torque constant) Kt=Ke for an ideal square wave motor : Gain  Gain=uav.motors(2).Ke_eq
  Saturation : Saturate  UpperLimit=uav.motors(2).current_limit  LowerLimit=0
  Sum : Sum  Inputs=|+-
  Electrical Torque : Outport  VectorParamsAs1DForOutWhenUnconnected=off
  current : Outport  Port=2  VectorParamsAs1DForOutWhenUnconnected=off
  wires:
  1/R/1 -> Saturation/1  "current i"
  Sum/1 -> 1/R/1
  Kt (Torque constant) Kt=Ke for an ideal square wave motor/1 -> Electrical Torque/1
  Ke (Torque constant)1/1 -> Sum/2
  ESC voltage/1 -> Sum/1
  w angular speed/1 -> Ke (Torque constant)1/1
  Saturation/1 -> Kt (Torque constant) Kt=Ke for an ideal square wave motor/1, current/1

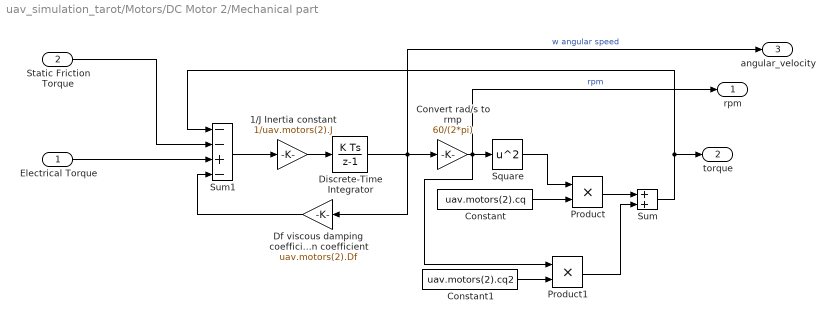
== system uav_simulation_tarot/Motors/DC Motor 2/Mechanical part ==
  Electrical Torque : Inport
  Static Friction Torque : Inport  Port=2
  1/J Inertia constant : Gain  Gain=1/uav.motors(2).J
  Constant : Constant  Value=uav.motors(2).cq
  Constant1 : Constant  Value=uav.motors(2).cq2
  Convert rad/s to rmp : Gain  Gain=60/(2*pi)
  "Df viscous damping coefficient Dynamic Friction coefficient " : Gain  Gain=uav.motors(2).Df
  Discrete-Time Integrator : DiscreteIntegrator  gainval=1  InitialCondition=sim_params.initial_conditions.w2  SampleTime=uav.dynamics_srate  ICPrevOutput=DiscIntNeverNeededParam  ICPrevScaledInput=DiscIntNeverNeededParam
  Product : Product
  Product1 : Product
  Square : Math  Operator=square  SaturateOnIntegerOverflow=on
  Sum : Sum
  Sum1 : Sum  Inputs=--+-
  rpm : Outport  VectorParamsAs1DForOutWhenUnconnected=off
  torque : Outport  Port=2
  angular_velocity : Outport  Port=3
  wires:
  1/J Inertia constant/1 -> Discrete-Time Integrator/1
  Static Friction Torque/1 -> Sum1/2
  "Df viscous damping coefficient Dynamic Friction coefficient "/1 -> Sum1/4
  Discrete-Time Integrator/1 -> angular_velocity/1, Convert rad/s to rmp/1, "Df viscous damping coefficient Dynamic Friction coefficient "/1  "w angular speed"
  Sum1/1 -> 1/J Inertia constant/1
  Electrical Torque/1 -> Sum1/3
  Sum/1 -> Sum1/1, torque/1
  Square/1 -> Product/1
  Constant/1 -> Product/2
  Product/1 -> Sum/1
  Constant1/1 -> Product1/2
  Convert rad/s to rmp/1 -> rpm/1, Product1/1, Square/1  "rpm"
  Product1/1 -> Sum/2

== system uav_simulation_tarot/Motors/DC Motor 3/Electrical part ==
  ESC voltage : Inport
  w angular speed : Inport  Port=2
  1/R : Gain  Gain=1/uav.motors(3).Req
  Ke (Torque constant)1 : Gain  Gain=uav.motors(3).Ke_eq
  Kt (Torque constant) Kt=Ke for an ideal square wave motor : Gain  Gain=uav.motors(3).Ke_eq
  Saturation : Saturate  UpperLimit=uav.motors(3).current_limit  LowerLimit=0
  Sum : Sum  Inputs=|+-
  Electrical Torque : Outport  VectorParamsAs1DForOutWhenUnconnected=off
  current : Outport  Port=2  VectorParamsAs1DForOutWhenUnconnected=off
  wires:
  1/R/1 -> Saturation/1  "current i"
  Sum/1 -> 1/R/1
  Kt (Torque constant) Kt=Ke for an ideal square wave motor/1 -> Electrical Torque/1
  Ke (Torque constant)1/1 -> Sum/2
  ESC voltage/1 -> Sum/1
  w angular speed/1 -> Ke (Torque constant)1/1
  Saturation/1 -> Kt (Torque constant) Kt=Ke for an ideal square wave motor/1, current/1

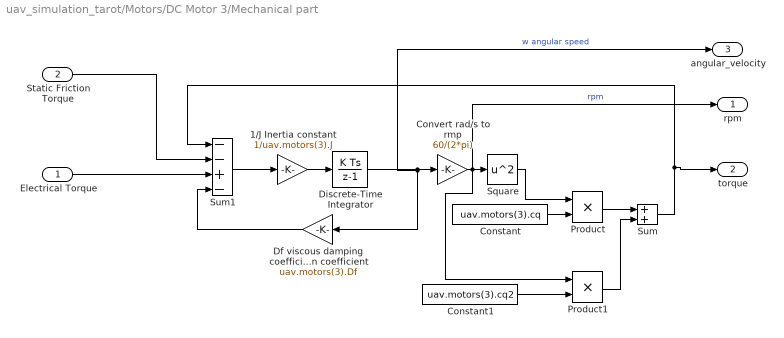
== system uav_simulation_tarot/Motors/DC Motor 3/Mechanical part ==
  Electrical Torque : Inport
  Static Friction Torque : Inport  Port=2
  1/J Inertia constant : Gain  Gain=1/uav.motors(3).J
  Constant : Constant  Value=uav.motors(3).cq
  Constant1 : Constant  Value=uav.motors(3).cq2
  Convert rad/s to rmp : Gain  Gain=60/(2*pi)
  "Df viscous damping coefficient Dynamic Friction coefficient " : Gain  Gain=uav.motors(3).Df
  Discrete-Time Integrator : DiscreteIntegrator  gainval=1  InitialCondition=sim_params.initial_conditions.w3  SampleTime=uav.dynamics_srate  ICPrevOutput=DiscIntNeverNeededParam  ICPrevScaledInput=DiscIntNeverNeededParam
  Product : Product
  Product1 : Product
  Square : Math  Operator=square  SaturateOnIntegerOverflow=on
  Sum : Sum
  Sum1 : Sum  Inputs=--+-
  rpm : Outport  VectorParamsAs1DForOutWhenUnconnected=off
  torque : Outport  Port=2
  angular_velocity : Outport  Port=3
  wires:
  1/J Inertia constant/1 -> Discrete-Time Integrator/1
  Static Friction Torque/1 -> Sum1/2
  "Df viscous damping coefficient Dynamic Friction coefficient "/1 -> Sum1/4
  Discrete-Time Integrator/1 -> angular_velocity/1, "Df viscous damping coefficient Dynamic Friction coefficient "/1, Convert rad/s to rmp/1  "w angular speed"
  Sum1/1 -> 1/J Inertia constant/1
  Electrical Torque/1 -> Sum1/3
  Sum/1 -> torque/1, Sum1/1
  Square/1 -> Product/1
  Constant/1 -> Product/2
  Product/1 -> Sum/1
  Constant1/1 -> Product1/2
  Convert rad/s to rmp/1 -> Product1/1, rpm/1, Square/1  "rpm"
  Product1/1 -> Sum/2

== system uav_simulation_tarot/Motors/DC Motor 4/Electrical part ==
  ESC voltage : Inport
  w angular speed : Inport  Port=2
  1/R : Gain  Gain=1/uav.motors(4).Req
  Ke (Torque constant)1 : Gain  Gain=uav.motors(4).Ke_eq
  Kt (Torque constant) Kt=Ke for an ideal square wave motor : Gain  Gain=uav.motors(4).Ke_eq
  Saturation : Saturate  UpperLimit=uav.motors(4).current_limit  LowerLimit=0
  Sum : Sum  Inputs=|+-
  Electrical Torque : Outport  VectorParamsAs1DForOutWhenUnconnected=off
  current : Outport  Port=2  VectorParamsAs1DForOutWhenUnconnected=off
  wires:
  1/R/1 -> Saturation/1  "current i"
  Sum/1 -> 1/R/1
  Kt (Torque constant) Kt=Ke for an ideal square wave motor/1 -> Electrical Torque/1
  Ke (Torque constant)1/1 -> Sum/2
  ESC voltage/1 -> Sum/1
  w angular speed/1 -> Ke (Torque constant)1/1
  Saturation/1 -> Kt (Torque constant) Kt=Ke for an ideal square wave motor/1, current/1

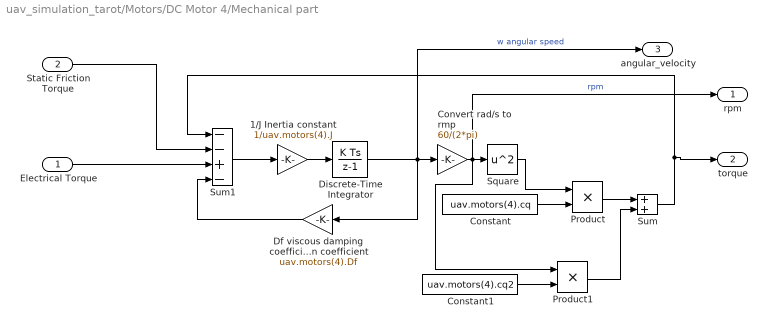
== system uav_simulation_tarot/Motors/DC Motor 4/Mechanical part ==
  Electrical Torque : Inport
  Static Friction Torque : Inport  Port=2
  1/J Inertia constant : Gain  Gain=1/uav.motors(4).J
  Constant : Constant  Value=uav.motors(4).cq
  Constant1 : Constant  Value=uav.motors(4).cq2
  Convert rad/s to rmp : Gain  Gain=60/(2*pi)
  "Df viscous damping coefficient Dynamic Friction coefficient " : Gain  Gain=uav.motors(4).Df
  Discrete-Time Integrator : DiscreteIntegrator  gainval=1  InitialCondition=sim_params.initial_conditions.w4  SampleTime=uav.dynamics_srate  ICPrevOutput=DiscIntNeverNeededParam  ICPrevScaledInput=DiscIntNeverNeededParam
  Product : Product
  Product1 : Product
  Square : Math  Operator=square  SaturateOnIntegerOverflow=on
  Sum : Sum
  Sum1 : Sum  Inputs=--+-
  rpm : Outport  VectorParamsAs1DForOutWhenUnconnected=off
  torque : Outport  Port=2
  angular_velocity : Outport  Port=3
  wires:
  1/J Inertia constant/1 -> Discrete-Time Integrator/1
  Static Friction Torque/1 -> Sum1/2
  "Df viscous damping coefficient Dynamic Friction coefficient "/1 -> Sum1/4
  Discrete-Time Integrator/1 -> angular_velocity/1, Convert rad/s to rmp/1, "Df viscous damping coefficient Dynamic Friction coefficient "/1  "w angular speed"
  Sum1/1 -> 1/J Inertia constant/1
  Electrical Torque/1 -> Sum1/3
  Sum/1 -> torque/1, Sum1/1
  Square/1 -> Product/1
  Constant/1 -> Product/2
  Product/1 -> Sum/1
  Constant1/1 -> Product1/2
  Convert rad/s to rmp/1 -> rpm/1, Product1/1, Square/1  "rpm"
  Product1/1 -> Sum/2

== system uav_simulation_tarot/Motors/DC Motor 5/Electrical part ==
  ESC voltage : Inport
  w angular speed : Inport  Port=2
  1/R : Gain  Gain=1/uav.motors(5).Req
  Ke (Torque constant)1 : Gain  Gain=uav.motors(5).Ke_eq
  Kt (Torque constant) Kt=Ke for an ideal square wave motor : Gain  Gain=uav.motors(5).Ke_eq
  Saturation : Saturate  UpperLimit=uav.motors(5).current_limit  LowerLimit=0
  Sum : Sum  Inputs=|+-
  Electrical Torque : Outport  VectorParamsAs1DForOutWhenUnconnected=off
  current : Outport  Port=2  VectorParamsAs1DForOutWhenUnconnected=off
  wires:
  1/R/1 -> Saturation/1  "current i"
  Sum/1 -> 1/R/1
  Kt (Torque constant) Kt=Ke for an ideal square wave motor/1 -> Electrical Torque/1
  Ke (Torque constant)1/1 -> Sum/2
  ESC voltage/1 -> Sum/1
  w angular speed/1 -> Ke (Torque constant)1/1
  Saturation/1 -> Kt (Torque constant) Kt=Ke for an ideal square wave motor/1, current/1

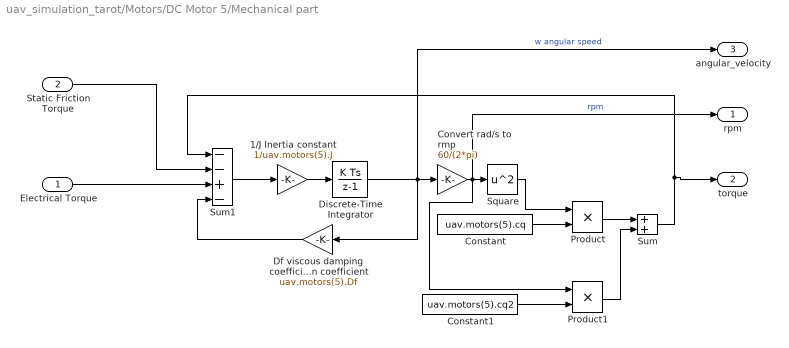
== system uav_simulation_tarot/Motors/DC Motor 5/Mechanical part ==
  Electrical Torque : Inport
  Static Friction Torque : Inport  Port=2
  1/J Inertia constant : Gain  Gain=1/uav.motors(5).J
  Constant : Constant  Value=uav.motors(5).cq
  Constant1 : Constant  Value=uav.motors(5).cq2
  Convert rad/s to rmp : Gain  Gain=60/(2*pi)
  "Df viscous damping coefficient Dynamic Friction coefficient " : Gain  Gain=uav.motors(5).Df
  Discrete-Time Integrator : DiscreteIntegrator  gainval=1  InitialCondition=sim_params.initial_conditions.w5  SampleTime=uav.dynamics_srate  ICPrevOutput=DiscIntNeverNeededParam  ICPrevScaledInput=DiscIntNeverNeededParam
  Product : Product
  Product1 : Product
  Square : Math  Operator=square  SaturateOnIntegerOverflow=on
  Sum : Sum
  Sum1 : Sum  Inputs=--+-
  rpm : Outport  VectorParamsAs1DForOutWhenUnconnected=off
  torque : Outport  Port=2
  angular_velocity : Outport  Port=3
  wires:
  1/J Inertia constant/1 -> Discrete-Time Integrator/1
  Static Friction Torque/1 -> Sum1/2
  "Df viscous damping coefficient Dynamic Friction coefficient "/1 -> Sum1/4
  Discrete-Time Integrator/1 -> angular_velocity/1, Convert rad/s to rmp/1, "Df viscous damping coefficient Dynamic Friction coefficient "/1  "w angular speed"
  Sum1/1 -> 1/J Inertia constant/1
  Electrical Torque/1 -> Sum1/3
  Sum/1 -> torque/1, Sum1/1
  Square/1 -> Product/1
  Constant/1 -> Product/2
  Product/1 -> Sum/1
  Constant1/1 -> Product1/2
  Convert rad/s to rmp/1 -> rpm/1, Product1/1, Square/1  "rpm"
  Product1/1 -> Sum/2

== system uav_simulation_tarot/Motors/DC Motor 6/Electrical part ==
  ESC voltage : Inport
  w angular speed : Inport  Port=2
  1/R : Gain  Gain=1/uav.motors(6).Req
  Ke (Torque constant)1 : Gain  Gain=uav.motors(6).Ke_eq
  Kt (Torque constant) Kt=Ke for an ideal square wave motor : Gain  Gain=uav.motors(6).Ke_eq
  Saturation : Saturate  UpperLimit=uav.motors(6).current_limit  LowerLimit=0
  Sum : Sum  Inputs=|+-
  Electrical Torque : Outport  VectorParamsAs1DForOutWhenUnconnected=off
  current : Outport  Port=2  VectorParamsAs1DForOutWhenUnconnected=off
  wires:
  1/R/1 -> Saturation/1  "current i"
  Sum/1 -> 1/R/1
  Kt (Torque constant) Kt=Ke for an ideal square wave motor/1 -> Electrical Torque/1
  Ke (Torque constant)1/1 -> Sum/2
  ESC voltage/1 -> Sum/1
  w angular speed/1 -> Ke (Torque constant)1/1
  Saturation/1 -> Kt (Torque constant) Kt=Ke for an ideal square wave motor/1, current/1

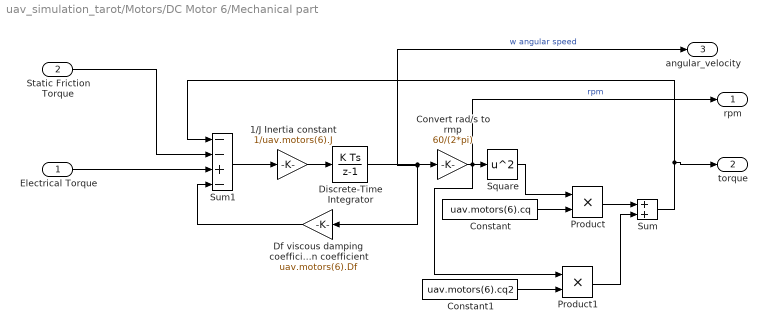
== system uav_simulation_tarot/Motors/DC Motor 6/Mechanical part ==
  Electrical Torque : Inport
  Static Friction Torque : Inport  Port=2
  1/J Inertia constant : Gain  Gain=1/uav.motors(6).J
  Constant : Constant  Value=uav.motors(6).cq
  Constant1 : Constant  Value=uav.motors(6).cq2
  Convert rad/s to rmp : Gain  Gain=60/(2*pi)
  "Df viscous damping coefficient Dynamic Friction coefficient " : Gain  Gain=uav.motors(6).Df
  Discrete-Time Integrator : DiscreteIntegrator  gainval=1  InitialCondition=sim_params.initial_conditions.w6  SampleTime=uav.dynamics_srate  ICPrevOutput=DiscIntNeverNeededParam  ICPrevScaledInput=DiscIntNeverNeededParam
  Product : Product
  Product1 : Product
  Square : Math  Operator=square  SaturateOnIntegerOverflow=on
  Sum : Sum
  Sum1 : Sum  Inputs=--+-
  rpm : Outport  VectorParamsAs1DForOutWhenUnconnected=off
  torque : Outport  Port=2
  angular_velocity : Outport  Port=3
  wires:
  1/J Inertia constant/1 -> Discrete-Time Integrator/1
  Static Friction Torque/1 -> Sum1/2
  "Df viscous damping coefficient Dynamic Friction coefficient "/1 -> Sum1/4
  Discrete-Time Integrator/1 -> angular_velocity/1, "Df viscous damping coefficient Dynamic Friction coefficient "/1, Convert rad/s to rmp/1  "w angular speed"
  Sum1/1 -> 1/J Inertia constant/1
  Electrical Torque/1 -> Sum1/3
  Sum/1 -> torque/1, Sum1/1
  Square/1 -> Product/1
  Constant/1 -> Product/2
  Product/1 -> Sum/1
  Constant1/1 -> Product1/2
  Convert rad/s to rmp/1 -> rpm/1, Product1/1, Square/1  "rpm"
  Product1/1 -> Sum/2

== system uav_simulation_tarot/Motors/DC Motor 7/Electrical part ==
  ESC voltage : Inport
  w angular speed : Inport  Port=2
  1/R : Gain  Gain=1/uav.motors(7).Req
  Ke (Torque constant)1 : Gain  Gain=uav.motors(7).Ke_eq
  Kt (Torque constant) Kt=Ke for an ideal square wave motor : Gain  Gain=uav.motors(7).Ke_eq
  Saturation : Saturate  UpperLimit=uav.motors(7).current_limit  LowerLimit=0
  Sum : Sum  Inputs=|+-
  Electrical Torque : Outport  VectorParamsAs1DForOutWhenUnconnected=off
  current : Outport  Port=2  VectorParamsAs1DForOutWhenUnconnected=off
  wires:
  1/R/1 -> Saturation/1  "current i"
  Sum/1 -> 1/R/1
  Kt (Torque constant) Kt=Ke for an ideal square wave motor/1 -> Electrical Torque/1
  Ke (Torque constant)1/1 -> Sum/2
  ESC voltage/1 -> Sum/1
  w angular speed/1 -> Ke (Torque constant)1/1
  Saturation/1 -> Kt (Torque constant) Kt=Ke for an ideal square wave motor/1, current/1

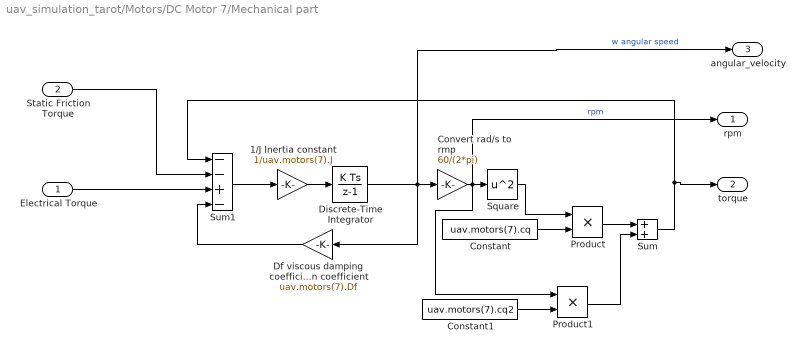
== system uav_simulation_tarot/Motors/DC Motor 7/Mechanical part ==
  Electrical Torque : Inport
  Static Friction Torque : Inport  Port=2
  1/J Inertia constant : Gain  Gain=1/uav.motors(7).J
  Constant : Constant  Value=uav.motors(7).cq
  Constant1 : Constant  Value=uav.motors(7).cq2
  Convert rad/s to rmp : Gain  Gain=60/(2*pi)
  "Df viscous damping coefficient Dynamic Friction coefficient " : Gain  Gain=uav.motors(7).Df
  Discrete-Time Integrator : DiscreteIntegrator  gainval=1  InitialCondition=sim_params.initial_conditions.w7  SampleTime=uav.dynamics_srate  ICPrevOutput=DiscIntNeverNeededParam  ICPrevScaledInput=DiscIntNeverNeededParam
  Product : Product
  Product1 : Product
  Square : Math  Operator=square  SaturateOnIntegerOverflow=on
  Sum : Sum
  Sum1 : Sum  Inputs=--+-
  rpm : Outport  VectorParamsAs1DForOutWhenUnconnected=off
  torque : Outport  Port=2
  angular_velocity : Outport  Port=3
  wires:
  1/J Inertia constant/1 -> Discrete-Time Integrator/1
  Static Friction Torque/1 -> Sum1/2
  "Df viscous damping coefficient Dynamic Friction coefficient "/1 -> Sum1/4
  Discrete-Time Integrator/1 -> "Df viscous damping coefficient Dynamic Friction coefficient "/1, angular_velocity/1, Convert rad/s to rmp/1  "w angular speed"
  Sum1/1 -> 1/J Inertia constant/1
  Electrical Torque/1 -> Sum1/3
  Sum/1 -> torque/1, Sum1/1
  Square/1 -> Product/1
  Constant/1 -> Product/2
  Product/1 -> Sum/1
  Constant1/1 -> Product1/2
  Convert rad/s to rmp/1 -> rpm/1, Product1/1, Square/1  "rpm"
  Product1/1 -> Sum/2

== system uav_simulation_tarot/Motors/DC Motor 8/Electrical part ==
  ESC voltage : Inport
  w angular speed : Inport  Port=2
  1/R : Gain  Gain=1/uav.motors(8).Req
  Ke (Torque constant)1 : Gain  Gain=uav.motors(8).Ke_eq
  Kt (Torque constant) Kt=Ke for an ideal square wave motor : Gain  Gain=uav.motors(8).Ke_eq
  Saturation : Saturate  UpperLimit=uav.motors(8).current_limit  LowerLimit=0
  Sum : Sum  Inputs=|+-
  Electrical Torque : Outport  VectorParamsAs1DForOutWhenUnconnected=off
  current : Outport  Port=2  VectorParamsAs1DForOutWhenUnconnected=off
  wires:
  1/R/1 -> Saturation/1  "current i"
  Sum/1 -> 1/R/1
  Kt (Torque constant) Kt=Ke for an ideal square wave motor/1 -> Electrical Torque/1
  Ke (Torque constant)1/1 -> Sum/2
  ESC voltage/1 -> Sum/1
  w angular speed/1 -> Ke (Torque constant)1/1
  Saturation/1 -> Kt (Torque constant) Kt=Ke for an ideal square wave motor/1, current/1
